simulink model "Adddata_Model"  (R2024b)
settings: Solver=VariableStepAuto  StartTime=0.0  StopTime=10.0  RelTol=1e-3
libraries: NSA_DEVS_SINKS x6, NSA_DEVS_LOGISTICS x5, NSA_DEVS_SOURCES x1
settings Model: Creator=david  LastModifiedBy=peter
settings RTWCC: GPUComputeCapability=3.5

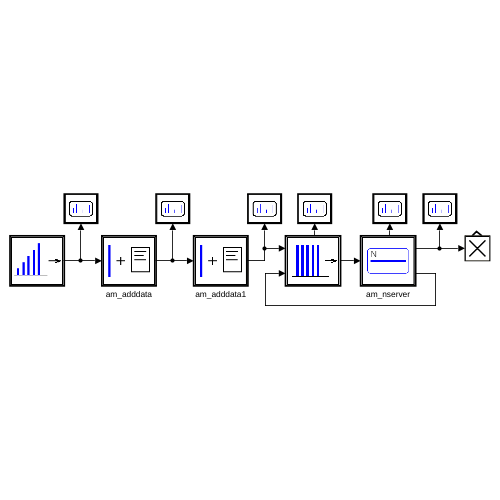
[thumbnail: Simulink's stored preview of the top-level diagram]
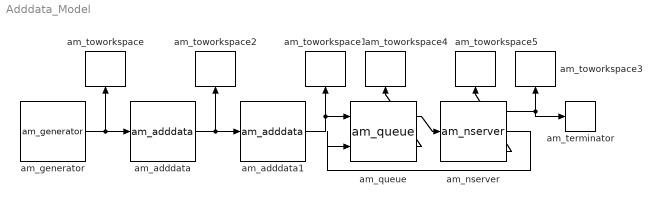
== system Adddata_Model ==
  am_adddata : NSA_DEVS_LOGISTICS/am_adddata  fields="[\"name\", \"age\"]"  values="[\"Krull\", \"36\"]"  numeric=[false, true]  infield="\"id\""  tau=[0,1]  debug=0
      settings: SourceProductName=Logistics
  am_adddata1 : NSA_DEVS_LOGISTICS/am_adddata  fields="[\"firstname\", \"weight\"]"  values="[\"Felix\", \"73\"]"  numeric=[false, true]  infield="\"id\""  tau=[0,1]  debug=0
      settings: SourceProductName=Logistics
  am_generator : NSA_DEVS_SOURCES/am_generator  tG=1  n0=1  nG=6  tD=[0,2]  debug=0
      settings: SourceProductName=Sources
  am_nserver : NSA_DEVS_LOGISTICS/am_nserver  N=3  tS=4.5  tsField="\"\""  tD=[0,2]  tau=[0,1]  debug=0
      settings: SourceProductName=Logistics
  am_queue : NSA_DEVS_LOGISTICS/am_queue  tD=[0,2]  tau=[0,1]  debug=0
      settings: SourceProductName=Logistics
  am_terminator : NSA_DEVS_LOGISTICS/am_terminator  tau=[0,1]  debug=0
      settings: SourceProductName=Logistics
  am_toworkspace : NSA_DEVS_SINKS/am_toworkspace  varname="\"genOut\""  t0=0  format="\"vector\""  tau=[0,3]  debug=0
      settings: SourceProductName=Sinks
  am_toworkspace1 : NSA_DEVS_SINKS/am_toworkspace  varname="\"data2Out\""  t0=0  format="\"vector\""  tau=[0,3]  debug=0
      settings: SourceProductName=Sinks
  am_toworkspace2 : NSA_DEVS_SINKS/am_toworkspace  varname="\"data1Out\""  t0=0  format="\"vector\""  tau=[0,3]  debug=0
      settings: SourceProductName=Sinks
  am_toworkspace3 : NSA_DEVS_SINKS/am_toworkspace  varname="\"srv2Out\""  t0=0  format="\"vector\""  tau=[0,3]  debug=0
      settings: SourceProductName=Sinks
  am_toworkspace4 : NSA_DEVS_SINKS/am_toworkspace  varname="\"nqOut\""  t0=0  format="\"vector\""  tau=[0,3]  debug=0
      settings: SourceProductName=Sinks
  am_toworkspace5 : NSA_DEVS_SINKS/am_toworkspace  varname="\"nsOut\""  t0=0  format="\"vector\""  tau=[0,5]  debug=0
      settings: SourceProductName=Sinks
  wires:
  am_generator/1 -> am_adddata/1, am_toworkspace/1
  am_adddata1/1 -> am_queue/1, am_toworkspace1/1
  am_adddata/1 -> am_adddata1/1, am_toworkspace2/1
  am_nserver/1 -> am_toworkspace3/1, am_terminator/1
  am_queue/1 -> am_nserver/1
  am_queue/2 -> am_toworkspace4/1
  am_nserver/3 -> am_toworkspace5/1
  am_nserver/2 -> am_queue/2
